simulink model "F_18"  (R2018a)
settings: Solver=VariableStepAuto  StartTime=0.0  StopTime=75  RelTol=1e-3
InitFcn:
  | vtol_param
  | F_f
  | F_f_b
StartFcn:
  | vtol_param
  | F_f
  | F_f_b
undefined symbols (not defined in the file or in its folder): P, PlotVtol
ContinueFcn:
  | FT2frfl
settings Model: Creator=sadam  LastModifiedBy=sadam

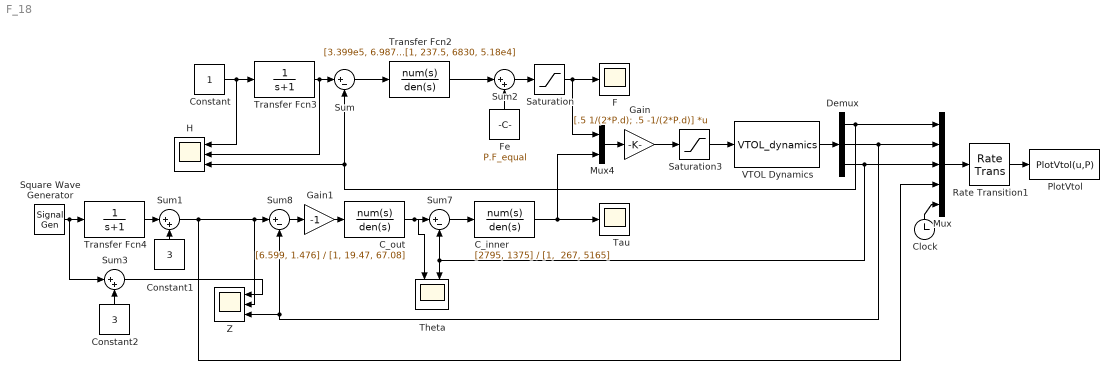
== system F_18 ==
  C_inner : TransferFcn  Numerator=[2795, 1375]  Denominator="[1,  267, 5165]"
  C_out : TransferFcn  Numerator=[6.599, 1.476]  Denominator=[1, 19.47, 67.08]
  Clock : Clock
  Constant : Constant
  Constant1 : Constant  Value=3
  Constant2 : Constant  Value=3
  Demux : Demux  Outputs=3
  F : Scope
  Fe : Constant  Value=P.F_equal
  Gain : Gain  Gain=[.5 1/(2*P.d); .5 -1/(2*P.d)]  Multiplication=Matrix(K*u)
  Gain1 : Gain  Gain=-1
  "H " : Scope  NumInputPorts=3
  Mux : Mux  Inputs=5
  Mux4 : Mux  Inputs=2
  "PlotVtol " : MATLABFcn  MATLABFcn=PlotVtol(u,P)  OutputDimensions=0
  Rate Transition1 : RateTransition  OutPortSampleTime=P.t_plot
  Saturation : Saturate  UpperLimit=P.Force_max  LowerLimit=-P.Force_max
  Saturation3 : Saturate  UpperLimit=P.Force_max  LowerLimit=-P.Force_max
  Square Wave Generator : SignalGenerator  WaveForm=square  Amplitude=2  Frequency=.05/2
  Sum : Sum  Inputs=|+-
  Sum1 : Sum  Inputs=|++
  Sum2 : Sum  Inputs=|++
  Sum3 : Sum  Inputs=|++
  Sum7 : Sum  Inputs=|+-
  Sum8 : Sum  Inputs=|+-
  Tau : Scope
  "Theta " : Scope  NumInputPorts=2
  Transfer Fcn2 : TransferFcn  Numerator=[3.399e5, 6.987e4]  Denominator=[1, 237.5, 6830, 5.18e4]
  Transfer Fcn3 : TransferFcn  Denominator=[1 1]
  Transfer Fcn4 : TransferFcn  Denominator=[1 1]
  VTOL Dynamics : S-Function  FunctionName=VTOL_dynamics  Parameters=P  SFunctionDeploymentMode=off  EnableBusSupport=off
  Z : Scope  NumInputPorts=3
  wires:
  Mux/1 -> Rate Transition1/1
  VTOL Dynamics/1 -> Demux/1
  Rate Transition1/1 -> "PlotVtol "/1
  Sum1/1 -> Z/2, Sum8/1, Mux/4
  Clock/1 -> Mux/5
  Demux/1 -> Mux/1, "H "/3, Sum/2
  Demux/2 -> Mux/2, Z/3, Sum8/2
  Demux/3 -> Mux/3, "Theta "/2, Sum7/2
  Saturation3/1 -> VTOL Dynamics/1
  Gain/1 -> Saturation3/1
  Mux4/1 -> Gain/1
  Sum2/1 -> Saturation/1
  Fe/1 -> Sum2/2
  Saturation/1 -> F/1, Mux4/1
  Constant1/1 -> Sum1/2
  Sum/1 -> Transfer Fcn2/1
  Transfer Fcn2/1 -> Sum2/1
  Constant/1 -> "H "/1, Transfer Fcn3/1
  Transfer Fcn3/1 -> "H "/2, Sum/1
  Sum7/1 -> C_inner/1
  C_inner/1 -> Mux4/2, Tau/1
  C_out/1 -> Sum7/1, "Theta "/1
  Transfer Fcn4/1 -> Sum1/1
  Square Wave Generator/1 -> Sum3/1, Transfer Fcn4/1
  Constant2/1 -> Sum3/2
  Sum3/1 -> Z/1
  Gain1/1 -> C_out/1
  Sum8/1 -> Gain1/1
